simulink model "Modelo9"  (R2020b)
settings: Solver=FixedStepAuto  StartTime=0.0  StopTime=inf  FixedStep=1e-2  MaxStep=1e-4  RelTol=1e-3
model workspace (MAT data in the model file):
  sensor_carga = Simulink.Parameter
  sensor_carga.DataType = 'auto'
  sensor_carga.Dimensions = [0 0]
values from neighbouring files (symbols this model uses):
  bcx = 1000e3    (= 1000000)    [Datos_simulacion.m]
  bcy = 500e3    (= 500000)    [Datos_simulacion.m]
  beq_tc = (bv_c+beq_cel)/Rw^2    (= 27000)    [Datos_simulacion.m]
  beq_ti = (b_h+beq_iel)/Rd^2    (= 28800)    [Datos_simulacion.m]
  bw = 30e3    (= 30000)    [Datos_simulacion.m]
  g = 9.80665    [Datos_simulacion.m]
  i_c = 15    [Datos_simulacion.m]
  i_i = 30    [Datos_simulacion.m]
  Kcd = Meq_c*polo_c*n    (= 472500)    [Datos_simulacion.m]
  Kci = Kcp*polo_c/n    (= 1938936.66179)    [Datos_simulacion.m]
  Kcp = Kcd*polo_c    (= 1513396.48861)    [Datos_simulacion.m]
  Kcy = 1.3e9    (= 1300000000)    [Datos_simulacion.m]
  Kid = Kcp*polo_i/n    (= 1815537.84919)    [Datos_simulacion.m]
  Kii = Meq_i*polo_i*n    (= 360000)    [Datos_simulacion.m]
  Kip = Kcd*polo_i    (= 1417080.12441)    [Datos_simulacion.m]
  Kw = 1800e3    (= 1800000)    [Datos_simulacion.m]
  Meq_c = m_c+Jeq_c/Rw^2    (= 59008)    [Datos_simulacion.m]
  Meq_i = m_h+Jeq_i/Rd^2    (= 48014.2222222)    [Datos_simulacion.m]
  Rd = 0.75    [Datos_simulacion.m]
  Rw = 0.5    [Datos_simulacion.m]
  Tau = 1e-3    (= 0.001)    [Datos_simulacion.m]
libraries: simulink x2, pid_lib x1, fuzblock x1, dspswit3 x1
(part 1 of 2)
settings Model: PauseTimes=6  Creator=GoniR  LastModifiedBy=GoniR
settings SolverCC: ConcurrentTasks=on  ZeroCrossAlgorithm=Adaptive  AutoInsertRateTranBlk=on
settings DebuggingCC: MaskedZcDiagnostic=none  IgnoredZcDiagnostic=none
settings HardwareCC: ProdHWDeviceType=AMD->x86-64 (Windows64)
settings SFSimCC: SimTargetLang=C++
settings ConfigComp: PLC_TargetIDE=codesys23

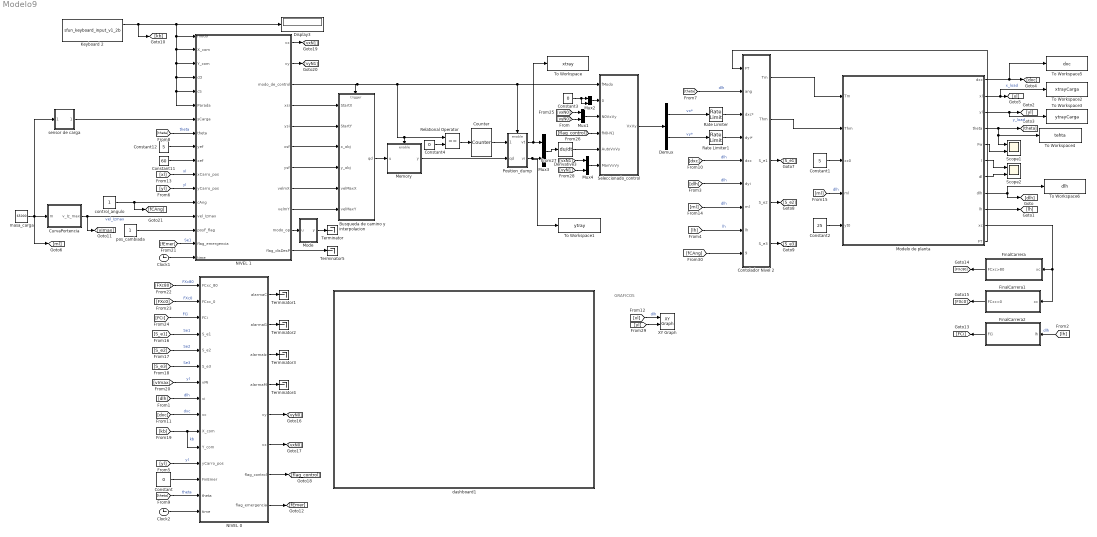
== system Modelo9 ==
  note: GRAFICOS
  Busqueda de camino y interpolacion : Subsystem
  Clock1 : Clock
  Clock2 : Clock
  Constant : Constant  Value=0
  Constant1 : Constant  Value=5
  Constant11 : Constant  Value=60
  Constant12 : Constant  Value=5
  Constant2 : Constant  Value=25
  Constant3 : Constant  Value=0
  Constant4 : Constant  Value=0
  Contolador Nivel 2 : Subsystem
  Counter : dspswit3/Counter  Direction=Up  CountEvent=Free running  CounterSize=User defined  MaxCount=100000  InitialCount=0  Output=Count  HitValue=32  ResetInput=on  SamplesPerFrame=1  Ts=-1  CntDtype=double  HitDtype=Logical
  CurvaPortencia : MATLAB Function  TreatAsAtomicUnit=on
  Demux : Demux  Outputs=2
  Derivative3 : Derivative
  Display3 : Display
  FinalCarrera : Subsystem
  FinalCarrera1 : Subsystem
  FinalCarrera2 : Subsystem
  Keyboard 2 : M-S-Function  FunctionName=sfun_keyboard_input_v1_2b  mask(Keyboard Input){}
      mask help: Keyboard Input
      mask Display: fprintf('Keyboard');
  Memory : Subsystem
  Mode : MATLAB Function  TreatAsAtomicUnit=on
  Modelo de planta : Subsystem
  Mux{1..4} (4 alike) : Mux  Inputs=2
  NIVEL 0 : Stateflow chart  TreatAsAtomicUnit=on
      settings: PortSchema="{\"entries\":[{\"content\":{\"sides\":[{\"content\":{\"connectorIds\":[\"In1\",\"In2\",\"In3\",\"In4\",\"In5\",\"In6\",\"In7\",\"In8\",\"In9\",\"In11\",\"In12\",\"In13\",\"In14\",\"In15\",\"In10\"]},\"type\":\"ConnectorPlacement.EquallySpacedRectSide\",\"uuid\":\"257bd8b2-e50d-4f94-a780-554a728b2489\"},{\"content\":{\"connectorIds\":[\"Out1\",\"Out2\",\"Out3\",\"Out4\",\"Out5\",\"Out6\",\"Out7\",\"Out8\"],\"side\":\"RIGHT\"},\"type\":\"ConnectorPlacement.EquallySpacedRectSide\",\"uuid\":\"e3415bb4-ca91-4503-b89e-6184bd1dfb63\"},{\"content\":{\"connectorIds\":[],\"side\":\"TOP\"},\"type\":\"ConnectorPlacement.EquallySpacedRectSide\",\"uuid\":\"9a32744b-d02f-467d-83f2-39baa82bdd9b\"},{\"content\":{\"connectorIds\":[],\"side\":\"HIDDEN\"},\"type\":\"ConnectorPlacement.EquallySpacedRectSide\",\"uuid\":\"21a6614f-2711-4cba-b5d3-48b2ed3c7fdc\"}]},\"type\":\"ConnectorPlacement.EquallySpacedConnector\",\"uuid\":\"64bd3217-fe30-40b0-9b87-0656394712b6\"}],\"packageUris\":[\"http://schema.mathworks.com/mf0/Connector/R2020b\"],\"version\":\"1.0\"}"
  NIVEL 1 : Stateflow chart  TreatAsAtomicUnit=on
      settings: PortSchema="{\"entries\":[{\"content\":{\"sides\":[{\"content\":{\"connectorIds\":[\"In13\",\"In1\",\"In2\",\"In5\",\"In6\",\"In10\",\"In7\",\"In14\",\"In3\",\"In4\",\"In9\",\"In12\",\"In8\",\"In15\",\"In17\",\"In16\",\"In11\"]},\"type\":\"ConnectorPlacement.EquallySpacedRectSide\",\"uuid\":\"1e4dd542-1771-4859-b91f-fc1cb250280a\"},{\"content\":{\"connectorIds\":[\"Out1\",\"Out2\",\"Out9\",\"Out7\",\"Out6\",\"Out8\",\"Out5\",\"Out4\",\"Out3\",\"Out10\",\"Out11\"],\"side\":\"RIGHT\"},\"type\":\"ConnectorPlacement.EquallySpacedRectSide\",\"uuid\":\"bb5e6521-c449-4a1c-9147-094c14f63665\"},{\"content\":{\"connectorIds\":[],\"side\":\"TOP\"},\"type\":\"ConnectorPlacement.EquallySpacedRectSide\",\"uuid\":\"54352a45-add1-4eb7-bb1e-2f57d731739f\"},{\"content\":{\"connectorIds\":[],\"side\":\"HIDDEN\"},\"type\":\"ConnectorPlacement.EquallySpacedRectSide\",\"uuid\":\"3e291a91-093a-4ab5-80ab-be4d5a353953\"}]},\"type\":\"ConnectorPlacement.EquallySpacedConnector\",\"uuid\":\"db8c49e8-a9b8-459f-b7fa-0d865c8e3061\"}],\"packageUris\":[\"http://schema.mathworks.com/mf0/Connector/R2020b\"],\"version\":\"1.0\"}"
  Position_dump : Subsystem
  Rate Limiter : RateLimiter  RisingSlewLimit=2  FallingSlewLimit=-2  SampleTimeMode=inherited
  Rate Limiter1 : RateLimiter  RisingSlewLimit=2  FallingSlewLimit=-2  SampleTimeMode=inherited
  Relational Operator : RelationalOperator  Operator===  OutDataTypeStr=boolean  RndMeth=Simplest
  Scope1 : Scope  NumInputPorts=2
  Scope2 : Scope  NumInputPorts=2
  Seleccionado_control : Subsystem
  Terminator{,1..5} (6 alike) : Terminator
  To Workspace : ToWorkspace  VariableName=xtray  SampleTime=-1
  To Workspace1 : ToWorkspace  VariableName=ytray  SampleTime=-1
  To Workspace2 : ToWorkspace  VariableName=xtrayCarga  SampleTime=-1
  To Workspace3 : ToWorkspace  VariableName=ytrayCarga  SampleTime=-1
  To Workspace4 : ToWorkspace  VariableName=tehta  SaveFormat=Timeseries  SampleTime=-1
  To Workspace5 : ToWorkspace  VariableName=dxc  SaveFormat=Timeseries  SampleTime=-1
  To Workspace6 : ToWorkspace  VariableName=dlh  SaveFormat=Timeseries  SampleTime=-1
  XY Graph : simulink/Sinks/XY Graph  xmin=0  xmax=80  ymin=0  ymax=60  st=-1
  control_angulo : Constant
  dashboard1 : Subsystem
  masa_carga : Constant  Value=65000
  pos_cambiada : Constant
  sensor de carga : Subsystem
  wires:
  Modelo de planta/2(xl) -> To Workspace2/1, [xl]  "x_load"
  Modelo de planta/3(yl) -> To Workspace3/1, [yl]  "y_load"
  Modelo de planta/7(dl) -> Scope2/2
  Modelo de planta/6(l) -> Scope2/1
  Modelo de planta/5(Fw) -> Scope1/2
  masa_carga/1 -> CurvaPortencia/1(m), [ml], sensor de carga/1(In1)
  Constant1/1 -> Modelo de planta/3(xc0)
  Constant2/1 -> Modelo de planta/5(yt0)
  Modelo de planta/4(theta) -> Scope1/1, To Workspace4/1, [theta]
  Memory/1(y) -> Position_dump/2(qd)
  Busqueda de camino y interpolacion/1(qd) -> Memory/1(u)
  Keyboard 2/1 -> NIVEL 1/2(Y_com), NIVEL 1/10(Parada), NIVEL 1/6(cS), NIVEL 1/5(cD), NIVEL 1/1(X_com), NIVEL 1/13(modo), Display3/1, [kb]
  Clock1/1 -> NIVEL 1/11(time)
  Constant11/1 -> NIVEL 1/4(xef)
  Constant12/1 -> NIVEL 1/3(yef)
  NIVEL 1/4(velmX) -> Busqueda de camino y interpolacion/5(velMaxX)
  NIVEL 1/3(velmY) -> Busqueda de camino y interpolacion/6(velMaxY)
  NIVEL 1/7(xsi) -> Busqueda de camino y interpolacion/1(StartX)
  NIVEL 1/6(ysi) -> Busqueda de camino y interpolacion/2(StartY)
  NIVEL 1/8(xsf) -> Busqueda de camino y interpolacion/3(x_obj)
  Position_dump/2(vi) -> To Workspace1/1, Mux3/2
  Demux/2 -> Rate Limiter1/1  "vy*"
  Demux/1 -> Rate Limiter/1  "vx*"
  control_angulo/1 -> NIVEL 1/8(cAng), [fCAng]
  NIVEL 1/10(modo_op) -> Mode/1(u)
  CurvaPortencia/1(v_Iz_max) -> NIVEL 1/15(vel_Izmax), [vImax]  "vel_Izmax"
  sensor de carga/1(Out1) -> NIVEL 1/7(sCarga)
  pos_cambiada/1 -> NIVEL 1/17(posF_flag)
  Mode/1(y) -> Terminator/1
  NIVEL 1/9(modo_de_control) -> Relational Operator/1, Memory/Enable, Seleccionado_control/1(fModo), Position_dump/Enable, Busqueda de camino y interpolacion/Trigger
  NIVEL 1/5(ysf) -> Busqueda de camino y interpolacion/4(y_obj)
  Rate Limiter/1 -> Contolador Nivel 2/3(dxc*)
  Modelo de planta/1(dxc) -> To Workspace5/1, [dxc]
  Modelo de planta/8(dlh) -> [dlh], To Workspace6/1
  Modelo de planta/9(lh) -> [lh]
  Contolador Nivel 2/1(Tm) -> Modelo de planta/1(Tm)
  Contolador Nivel 2/2(Thm) -> Modelo de planta/2(Thm)
  Rate Limiter1/1 -> Contolador Nivel 2/4(dyi*)
  Modelo de planta/10(xc) -> FinalCarrera1/1(xc), FinalCarrera/1(xc)
  Clock2/1 -> NIVEL 0/10(time)
  NIVEL 0/1(alarmaC) -> Terminator1/1
  NIVEL 0/2(alarmaG) -> Terminator2/1
  NIVEL 0/3(alarmaIz) -> Terminator3/1
  NIVEL 0/4(alarmaM) -> Terminator4/1
  Mux3/1 -> Derivative3/1
  Constant/1 -> NIVEL 0/14(FinEmer)
  NIVEL 0/8(flag_emergencia) -> [fEmer]
  Constant3/1 -> Mux2/1, Mux2/2
  Position_dump/1(vt) -> To Workspace/1, Mux3/1
  Constant4/1 -> Relational Operator/2
  Relational Operator/1 -> Counter/1
  Counter/1 -> Position_dump/1(counter)
  [dlh] -> Contolador Nivel 2/6(dyi)  "dlh"
  [dlh] -> NIVEL 0/8(vi)  "dlh"
  [lh] -> FinalCarrera2/1(lh)  "dlh"
  [lh] -> Contolador Nivel 2/8(lh)  "lh"
  [yl] -> NIVEL 0/13(yCarro_pos)  "yl"
  [yl] -> NIVEL 1/12(yCarro_pos)  "yl"
  [theta] -> Contolador Nivel 2/2(ang)  "dlh"
  [theta] -> NIVEL 0/15(theta)  "theta"
  [dxc] -> Contolador Nivel 2/5(dxc)  "dlh"
  [dxc] -> NIVEL 0/9(vc)  "dxc"
  [xl] -> XY Graph/1  "dlh"
  [xl] -> NIVEL 1/9(xCarro_pos)  "xl"
  [ml] -> Contolador Nivel 2/7(ml)  "dlh"
  [ml] -> Modelo de planta/4(ml)  "dlh"
  Contolador Nivel 2/3(S_e1) -> [S_e1]
  Contolador Nivel 2/4(S_e2) -> [S_e2]
  Contolador Nivel 2/5(S_e3) -> [S_e3]
  [S_e1] -> NIVEL 0/4(S_e1)  "Se1"
  [S_e2] -> NIVEL 0/5(S_e2)  "Se2"
  [S_e3] -> NIVEL 0/6(S_e3)  "Se3"
  [theta] -> NIVEL 1/14(theta)  "theta"
  [kb] -> NIVEL 0/12(Y_com), NIVEL 0/11(X_com)  "kb"
  [vImax] -> NIVEL 0/7(vMi)  "yl"
  [fEmer] -> NIVEL 1/16(flag_emergencia)  "Se1"
  FinalCarrera2/1(FCi) -> [FCi]
  FinalCarrera1/1(FCxc<0) -> [FXc0]
  FinalCarrera/1(FCxc>80) -> [FXc80]
  [FCi] -> NIVEL 0/3(FCi)  "FCi"
  [FXc0] -> NIVEL 0/2(FCxc_0)  "FXc0"
  [FXc80] -> NIVEL 0/1(FCxc_80)  "FXc80"
  NIVEL 0/5(vy) -> [vyN0]
  NIVEL 0/6(vx) -> [vxN0]
  [vyN0] -> Mux1/2
  [vxN0] -> Mux1/1
  NIVEL 0/7(flag_control) -> [flag_control]
  NIVEL 1/1(vx) -> [vxN1]
  NIVEL 1/2(vy) -> [vyN1]
  [vxN1] -> Mux4/1
  [vyN1] -> Mux4/2
  Mux2/1 -> Seleccionado_control/2(0)
  Mux1/1 -> Seleccionado_control/3(N0VxVy)
  [flag_control] -> Seleccionado_control/4(fN0-N1)
  Derivative3/1 -> Seleccionado_control/5(AutoVxVy)
  Mux4/1 -> Seleccionado_control/6(ManVxVy)
  Seleccionado_control/1(VxVy) -> Demux/1
  [yl] -> XY Graph/2
  NIVEL 1/11(flag_disDesP) -> Terminator5/1
  [fCAng] -> Contolador Nivel 2/9(fCAng)
  Modelo de planta/11(FT) -> Contolador Nivel 2/1(FT)

== system Modelo9/Busqueda de camino y interpolacion ==
  StartX : Inport
  StartY : Inport  Port=2
  x_obj : Inport  Port=3
  y_obj : Inport  Port=4
  velMaxX : Inport  Port=5
  velMaxY : Inport  Port=6
  Trigger : TriggerPort  VariantControl=Variant  PortDimensions=1
  Astart : MATLAB Function  TreatAsAtomicUnit=on
  Interpolador : MATLAB Function  TreatAsAtomicUnit=on
  qd : Outport
  wires:
  StartX/1 -> Astart/1(StartX)
  y_obj/1 -> Astart/4(y_obj)
  x_obj/1 -> Astart/3(x_obj)
  StartY/1 -> Astart/2(StartY)
  Astart/1(OptimalPath2) -> Interpolador/1(wayPoints)
  velMaxX/1 -> Interpolador/2(velMaxX)
  velMaxY/1 -> Interpolador/3(velMaxY)
  Interpolador/1(q) -> qd/1

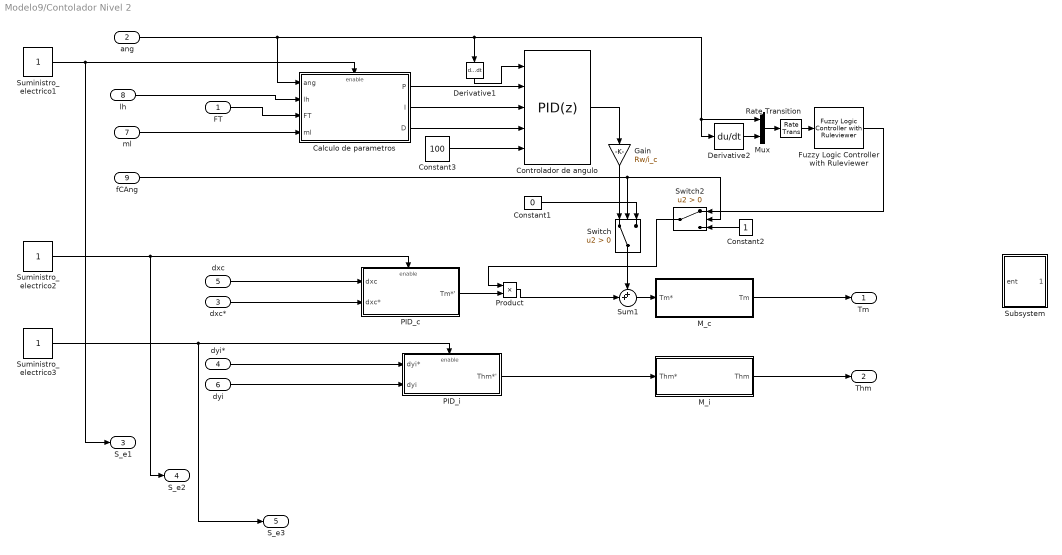
== system Modelo9/Contolador Nivel 2 ==
  FT : Inport
  ang : Inport  Port=2
  dxc* : Inport  Port=3
  dyi* : Inport  Port=4
  dxc : Inport  Port=5
  dyi : Inport  Port=6
  ml : Inport  Port=7
  lh : Inport  Port=8
  fCAng : Inport  Port=9
  Calculo de parametros : Subsystem
  Constant1 : Constant  Value=0
  Constant2 : Constant
  Constant3 : Constant  Value=100
  Controlador de angulo : pid_lib/PID Controller  Controller=PID  Form=Parallel  TimeDomain=Discrete-time  UseExternalTs=off  SampleTime=0.01  IntegratorMethod=Forward Euler  FilterMethod=Forward Euler  ControllerParametersSource=external  P=1  I=1  D=0  UseFilter=on  N=100  TunerSelectOption=Transfer Function Based (PID Tuner App)  InitialConditionSource=internal  InitialConditionForIntegrator=0  InitialConditionForFilter=0  DifferentiatorICPrevScaledInput=0  ExternalReset=none  TrackingMode=off  Kt=1  LimitOutput=off  SatLimitsSource=internal  UpperSaturationLimit=inf  LowerSaturationLimit=-inf  LinearizeAsGain=on  AntiWindupMode=none  Kb=1  POutMin=[]  POutMax=[]  IOutMin=[]  IOutMax=[]  DOutMin=[]  DOutMax=[]  NOutMin=[]  NOutMax=[]  SumOutMin=[]  SumOutMax=[]  SaturationOutMin=[]  SaturationOutMax=[]  PParamMin=[]  PParamMax=[]  IParamMin=[]  IParamMax=[]  DParamMin=[]  DParamMax=[]  NParamMin=[]  NParamMax=[]  KbParamMin=[]  KbParamMax=[]  KtParamMin=[]  KtParamMax=[]  KbOutMin=[]  KbOutMax=[]  KtOutMin=[]  KtOutMax=[]  IntegratorOutMin=[]  IntegratorOutMax=[]  FilterOutMin=[]  FilterOutMax=[]  SumI1OutMin=[]  SumI1OutMax=[]  SumI2OutMin=[]  SumI2OutMax=[]  SumI3OutMin=[]  SumI3OutMax=[]  SumI4OutMin=[]  SumI4OutMax=[]  SumDOutMin=[]  SumDOutMax=[]  DifferentiatorOutMin=[]  DifferentiatorOutMax=[]  FilterDiffOutCoefMin=[]  FilterDiffOutCoefMax=[]  ReciprocalOutMin=[]  ReciprocalOutMax=[]  SumDenOutMin=[]  SumDenOutMax=[]  SumNumOutMin=[]  SumNumOutMax=[]  DivideOutMin=[]  DivideOutMax=[]  UdiffTsProdOutMin=[]  UdiffTsProdOutMax=[]  NTsProdOutMin=[]  NTsProdOutMax=[]  UintegralTsProdOutMin=[]  UintegralTsProdOutMax=[]  UngainTsProdOutMin=[]  UngainTsProdOutMax=[]  IntegratorContinuousStateAttributes=''  IntegratorStateMustResolveToSignalObject=off  IntegratorRTWStateStorageClass=Auto  FilterContinuousStateAttributes=''  FilterStateMustResolveToSignalObject=off  FilterRTWStateStorageClass=Auto  ParallelPVariant=ExternalParameters  IdealPVariant=Disabled  IVariant=ExternalParameters  DVariant=ExternalParameters  IntegratorVariant=Discrete  SatVariant=Disabled  AWVariant=Passthrough  PCopyVariant=Disabled  TRVariant=Disabled  FdbkBlocksVariant=Forward  IdealPFdbkVariant=Disabled  SatFdbkVariant=Disabled  DerivativeFilterVariant=ForwardEulerFilter  NVariant=ExternalParameters  NCopyVariant=Disabled  FilterICVariant=InternalICsFilter  IntegratorICVariant=InternalICs  ExternalResetVariant=Disabled  TRSumVariant=Passthrough  SumFdbkVariant=Disabled  SumVariant=Sum_PID  TsampFilterVariant=InternalTs  TsampNgainVariant=Passthrough  TsampIntegralVariant=Passthrough  ExternalSaturationOutDataTypeStr=Inherit: Same as second input
  Derivative1 : Derivative
  Derivative2 : Derivative
  Fuzzy Logic Controller with Ruleviewer : fuzblock/Fuzzy Logic  Controller  with Ruleviewer  fismatrix=Control2  Ts=0.5
  Gain : Gain  Gain=Rw/i_c
  M_c : Subsystem
  M_i : Subsystem
  Mux : Mux  Inputs=2
  PID_c : Subsystem
  PID_i : Subsystem
  Product : Product
  Rate Transition : RateTransition  OutPortSampleTime=0.01
  Subsystem : Subsystem
  Sum1 : Sum  Inputs=++|
  Suministro_electrico1 : Constant
  Suministro_electrico2 : Constant
  Suministro_electrico3 : Constant
  Switch : Switch  Criteria=u2 > Threshold
  Switch2 : Switch  Criteria=u2 > Threshold
  Tm : Outport
  Thm : Outport  Port=2
  S_e1 : Outport  Port=3
  S_e2 : Outport  Port=4
  S_e3 : Outport  Port=5
  wires:
  Constant3/1 -> Controlador de angulo/5
  Fuzzy Logic Controller with Ruleviewer/1 -> Switch2/1
  Rate Transition/1 -> Fuzzy Logic Controller with Ruleviewer/1
  M_i/1(Thm) -> Thm/1
  Calculo de parametros/1(P) -> Controlador de angulo/2
  PID_i/1(Thm*') -> M_i/1(Thm*)
  Calculo de parametros/3(D) -> Controlador de angulo/4
  Calculo de parametros/2(I) -> Controlador de angulo/3
  ml/1 -> Calculo de parametros/4(ml)
  Mux/1 -> Rate Transition/1
  PID_c/1(Tm*') -> Product/2
  Sum1/1 -> M_c/1(Tm*)
  M_c/1(Tm) -> Tm/1
  dxc*/1 -> PID_c/2(dxc*)
  lh/1 -> Calculo de parametros/2(lh)
  dyi*/1 -> PID_i/1(dyi*)
  dxc/1 -> PID_c/1(dxc)
  dyi/1 -> PID_i/2(dyi)
  Derivative2/1 -> Mux/2
  Suministro_electrico1/1 -> S_e1/1, Calculo de parametros/Enable
  Suministro_electrico3/1 -> PID_i/Enable, S_e3/1
  Suministro_electrico2/1 -> S_e2/1, PID_c/Enable
  Switch/1 -> Sum1/1
  fCAng/1 -> Switch2/2, Switch/2
  Constant1/1 -> Switch/3
  Controlador de angulo/1 -> Gain/1
  Constant2/1 -> Switch2/3
  Switch2/1 -> Product/1
  Product/1 -> Sum1/2
  FT/1 -> Calculo de parametros/3(FT)
  Gain/1 -> Switch/1
  ang/1 -> Derivative2/1, Mux/1, Derivative1/1, Calculo de parametros/1(ang)
  Derivative1/1 -> Controlador de angulo/1

== system Modelo9/FinalCarrera ==
  xc : Inport
  Constant : Constant
  Constant1 : Constant  Value=0
  Switch : Switch  Criteria=u2 > Threshold  Threshold=80
  FCxc>80 : Outport
  wires:
  Constant/1 -> Switch/1
  Constant1/1 -> Switch/3
  Switch/1 -> FCxc>80/1
  xc/1 -> Switch/2

== system Modelo9/FinalCarrera1 ==
  xc : Inport
  Constant : Constant
  Constant1 : Constant  Value=0
  Gain : Gain  Gain=-1
  Switch : Switch  Criteria=u2 > Threshold
  FCxc<0 : Outport
  wires:
  Constant/1 -> Switch/1
  Constant1/1 -> Switch/3
  Switch/1 -> FCxc<0/1
  xc/1 -> Gain/1
  Gain/1 -> Switch/2

== system Modelo9/FinalCarrera2 ==
  lh : Inport
  Constant : Constant
  Constant1 : Constant  Value=0
  Gain : Gain  Gain=-1
  Switch : Switch
  FCi : Outport
  wires:
  Constant/1 -> Switch/1
  Constant1/1 -> Switch/3
  Switch/1 -> FCi/1
  lh/1 -> Gain/1
  Gain/1 -> Switch/2

== system Modelo9/Memory ==
  u : Inport
  Enable : EnablePort
  y : Outport
  wires:
  u/1 -> y/1

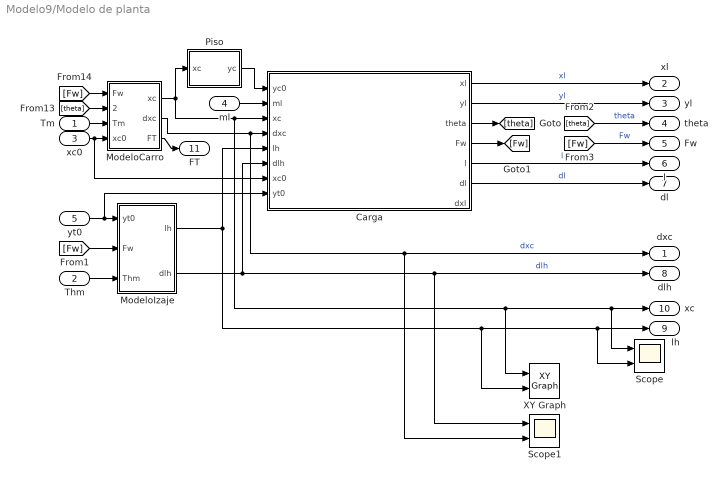
== system Modelo9/Modelo de planta ==
  Tm : Inport
  Thm : Inport  Port=2
  xc0 : Inport  Port=3
  ml : Inport  Port=4
  yt0 : Inport  Port=5
  Carga : Subsystem
  ModeloCarro : Subsystem
  ModeloIzaje : Subsystem
  Piso : Subsystem
  Scope : Scope  NumInputPorts=2
  Scope1 : Scope  NumInputPorts=2
  XY Graph : simulink/Sinks/XY Graph  xmin=0  xmax=80  ymin=0  ymax=60  st=-1
  dxc : Outport
  xl : Outport  Port=2
  yl : Outport  Port=3
  theta : Outport  Port=4
  Fw : Outport  Port=5
  l : Outport  Port=6
  dl : Outport  Port=7
  dlh : Outport  Port=8
  lh : Outport  Port=9
  xc : Outport  Port=10
  FT : Outport  Port=11
  wires:
  ModeloCarro/1(xc) -> XY Graph/1, Scope/1, xc/1, Carga/3(xc), Piso/1(xc)
  ModeloCarro/2(dxc) -> Scope1/2, dxc/1, Carga/4(dxc)  "dxc"
  ModeloIzaje/1(lh) -> XY Graph/2, Scope/2, lh/1, Carga/5(lh)
  ModeloIzaje/2(dlh) -> Carga/6(dlh), Scope1/1, dlh/1  "dlh"
  Carga/4(Fw) -> [Fw]
  [Fw] -> ModeloCarro/1(Fw)
  [Fw] -> ModeloIzaje/2(Fw)
  Carga/3(theta) -> [theta]
  [theta] -> ModeloCarro/2(theta)
  Carga/1(xl) -> xl/1  "xl"
  Carga/2(yl) -> yl/1  "yl"
  Carga/5(l) -> l/1  "l"
  Carga/6(dl) -> dl/1  "dl"
  [theta] -> theta/1  "theta"
  [Fw] -> Fw/1  "Fw"
  ml/1 -> Carga/2(ml)
  Thm/1 -> ModeloIzaje/3(Thm)
  Tm/1 -> ModeloCarro/3(Tm)
  Piso/1(yc) -> Carga/1(yc0)
  yt0/1 -> Carga/8(yt0), ModeloIzaje/1(yt0)
  xc0/1 -> Carga/7(xc0), ModeloCarro/4(xc0)
  ModeloCarro/3(FT) -> FT/1

== system Modelo9/Position_dump ==
  counter : Inport
  qd : Inport  Port=2
  Enable : EnablePort  PropagateVarSize=During execution
  MATLAB Function : MATLAB Function  TreatAsAtomicUnit=on
  Rate Transition : RateTransition
  Scope1 : Scope
  vt : Outport
  vi : Outport  Port=2
  wires:
  MATLAB Function/1(vt) -> vt/1
  MATLAB Function/2(vi) -> vi/1
  qd/1 -> MATLAB Function/1(qd)
  Rate Transition/1 -> Scope1/1, MATLAB Function/2(cont_i)
  counter/1 -> Rate Transition/1

== system Modelo9/Seleccionado_control ==
  fModo : Inport
  0 : Inport  Port=2
  N0VxVy : Inport  Port=3
  fN0-N1 : Inport  Port=4
  AutoVxVy : Inport  Port=5
  ManVxVy : Inport  Port=6
  AutoOn/Off : Switch  Criteria=u2 > Threshold
  M_o_A : Switch  Criteria=u2 > Threshold
  N0_o_N1 : Switch  Criteria=u2 > Threshold
  VxVy : Outport
  wires:
  AutoOn/Off/1 -> M_o_A/1
  N0_o_N1/1 -> VxVy/1
  M_o_A/1 -> N0_o_N1/3
  ManVxVy/1 -> M_o_A/3
  AutoVxVy/1 -> AutoOn/Off/1
  fModo/1 -> AutoOn/Off/2, M_o_A/2
  0/1 -> AutoOn/Off/3
  fN0-N1/1 -> N0_o_N1/2
  N0VxVy/1 -> N0_o_N1/1

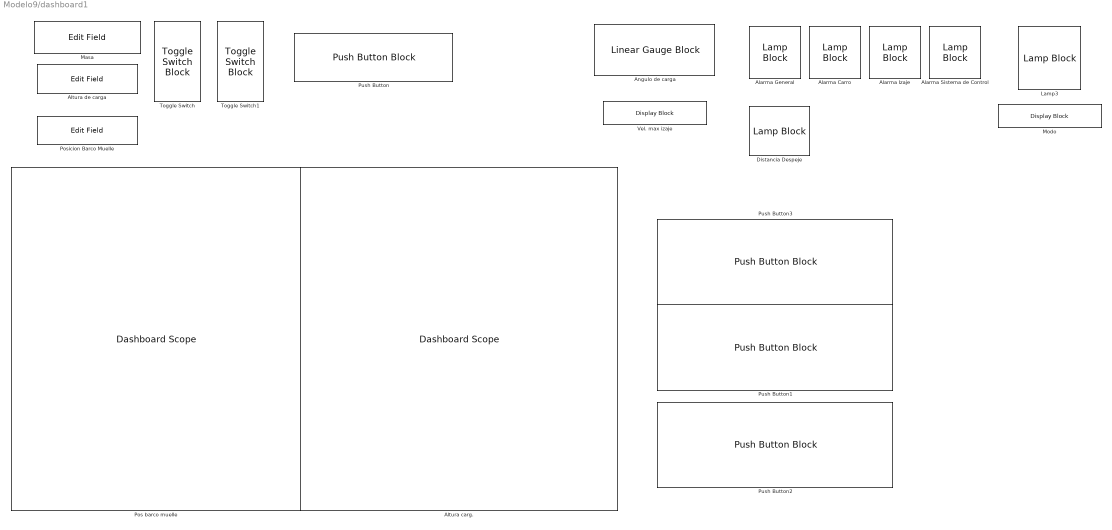
== system Modelo9/dashboard1 ==
  Alarma Carro : LampBlock
  Alarma General : LampBlock
  Alarma Izaje : LampBlock
  Alarma Sistema de Control : LampBlock
  Altura carg. : DashboardScope
  Altura de carga : EditField  LabelPosition=Hide  ShowInitialText=on  Alignment=Center
  Angulo de carga : LinearGaugeBlock  LabelPosition=Hide  ScaleMin=-0.15  ScaleMax=0.15
  Distancia Despeje : LampBlock
  Lamp3 : LampBlock  LabelPosition=Bottom
  Masa : EditField  LabelPosition=Hide  ShowInitialText=on  Alignment=Center
  Modo : DisplayBlock  LabelPosition=Hide  Format=short  Transparency=1
  Pos barco muelle : DashboardScope
  Posicion Barco Muelle : EditField  LabelPosition=Hide  ShowInitialText=on  Alignment=Center
  Push Button : PushButtonBlock  ButtonText=Fin Emergencia
  Push Button1 : PushButtonBlock  ButtonText=Falla Microcontrolador1  OnValue=0
  Push Button2 : PushButtonBlock  ButtonText=Falla Microcontrolador3  OnValue=0
  Push Button3 : PushButtonBlock  ButtonText=Falla Microcontrolador2  OnValue=0
  Toggle Switch : ToggleSwitchBlock
      settings: Values={{'Off', 'On'}, [0 1]}
  Toggle Switch1 : ToggleSwitchBlock
      settings: Values={{'Sin Cambiar', 'Cambiada'}, [0 1]}
  Vel. max izaje : DisplayBlock  LabelPosition=Hide  Format=short  Transparency=1

== system Modelo9/sensor de carga ==
  In1 : Inport
  Constant5 : Constant
  Constant6 : Constant  Value=0
  Switch1 : Switch  Criteria=u2 > Threshold  Threshold=15000
  Out1 : Outport
  wires:
  Constant5/1 -> Switch1/1
  Constant6/1 -> Switch1/3
  Switch1/1 -> Out1/1
  In1/1 -> Switch1/2

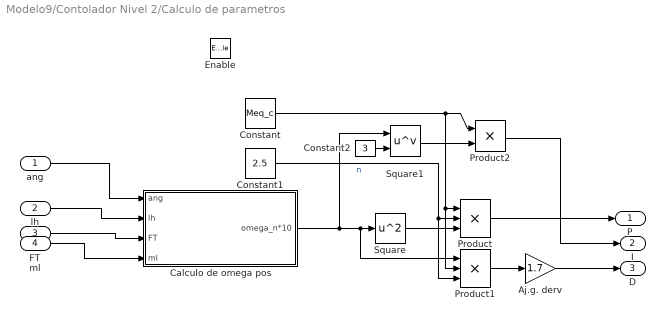
== system Modelo9/Contolador Nivel 2/Calculo de parametros ==
  ang : Inport
  lh : Inport  Port=2
  FT : Inport  Port=3
  ml : Inport  Port=4
  Enable : EnablePort
  Aj.g. derv : Gain  Gain=1.7
  Calculo de omega pos : Subsystem
  Constant : Constant  Value=Meq_c
  Constant1 : Constant  Value=2.5
  Constant2 : Constant  Value=3
  Product : Product  Inputs=3
  Product1 : Product  Inputs=3
  Product2 : Product
  Square : Math  Operator=square  SaturateOnIntegerOverflow=on
  Square1 : Math  Operator=pow  SaturateOnIntegerOverflow=on
  P : Outport
  I : Outport  Port=2
  D : Outport  Port=3
  wires:
  lh/1 -> Calculo de omega pos/2(lh)
  Constant1/1 -> Product/2, Product1/3  "n"
  Calculo de omega pos/1(omega_n*10) -> Square1/1, Product1/1, Square/1
  Constant/1 -> Product1/2, Product/1, Product2/1
  Product/1 -> P/1
  Product1/1 -> Aj.g. derv/1
  Square/1 -> Product/3
  ml/1 -> Calculo de omega pos/4(ml)
  Product2/1 -> I/1
  Aj.g. derv/1 -> D/1
  Square1/1 -> Product2/2
  Constant2/1 -> Square1/2
  FT/1 -> Calculo de omega pos/3(FT)
  ang/1 -> Calculo de omega pos/1(ang)

== system Modelo9/Contolador Nivel 2/M_c ==
  Tm* : Inport
  Transfer Fcn : TransferFcn  Denominator=[0.05 1]
  Tm : Outport
  wires:
  Tm*/1 -> Transfer Fcn/1
  Transfer Fcn/1 -> Tm/1

== system Modelo9/Contolador Nivel 2/M_i ==
  Thm* : Inport
  Transfer Fcn : TransferFcn  Denominator=[Tau 1]
  Thm : Outport
  wires:
  Thm*/1 -> Transfer Fcn/1
  Transfer Fcn/1 -> Thm/1

== system Modelo9/Contolador Nivel 2/PID_c ==
  dxc : Inport
  dxc* : Inport  Port=2
  Enable : EnablePort
  Gain : Gain  Gain=Kcp
  Gain1 : Gain  Gain=Kci
  Gain2 : Gain  Gain=Kcd
  Integrator : Integrator
  Integrator1 : Integrator
  Sum : Sum  Inputs=|+-
  Sum1 : Sum  Inputs=+++
  Tm*' : Outport
  wires:
  dxc*/1 -> Sum/1
  dxc/1 -> Sum/2
  Sum1/1 -> Tm*'/1
  Gain2/1 -> Sum1/3
  Gain/1 -> Sum1/2
  Gain1/1 -> Sum1/1
  Sum/1 -> Integrator1/1, Gain2/1
  Integrator1/1 -> Integrator/1, Gain/1
  Integrator/1 -> Gain1/1

== system Modelo9/Contolador Nivel 2/PID_i ==
  dyi* : Inport
  dyi : Inport  Port=2
  Enable : EnablePort
  Gain : Gain  Gain=Kip
  Gain1 : Gain  Gain=Kii
  Gain2 : Gain  Gain=Kid
  Integrator : Integrator
  Integrator1 : Integrator
  Sum : Sum  Inputs=|+-
  Sum1 : Sum  Inputs=+++
  Thm*' : Outport
  wires:
  dyi*/1 -> Sum/1
  dyi/1 -> Sum/2
  Sum1/1 -> Thm*'/1
  Gain2/1 -> Sum1/3
  Gain/1 -> Sum1/2
  Gain1/1 -> Sum1/1
  Sum/1 -> Integrator/1, Gain2/1
  Integrator/1 -> Integrator1/1, Gain/1
  Integrator1/1 -> Gain1/1

== system Modelo9/Contolador Nivel 2/Subsystem ==
  ent : Inport
  5secTimer : Subsystem
  Delay : Delay
  inv : Subsystem
  timer : Outport
  wires:
  ent/1 -> inv/1(ent)
  inv/1(inv) -> Delay/1, 5secTimer/Enable
  5secTimer/1(Out1) -> timer/1
  Delay/1 -> 5secTimer/1(In1)

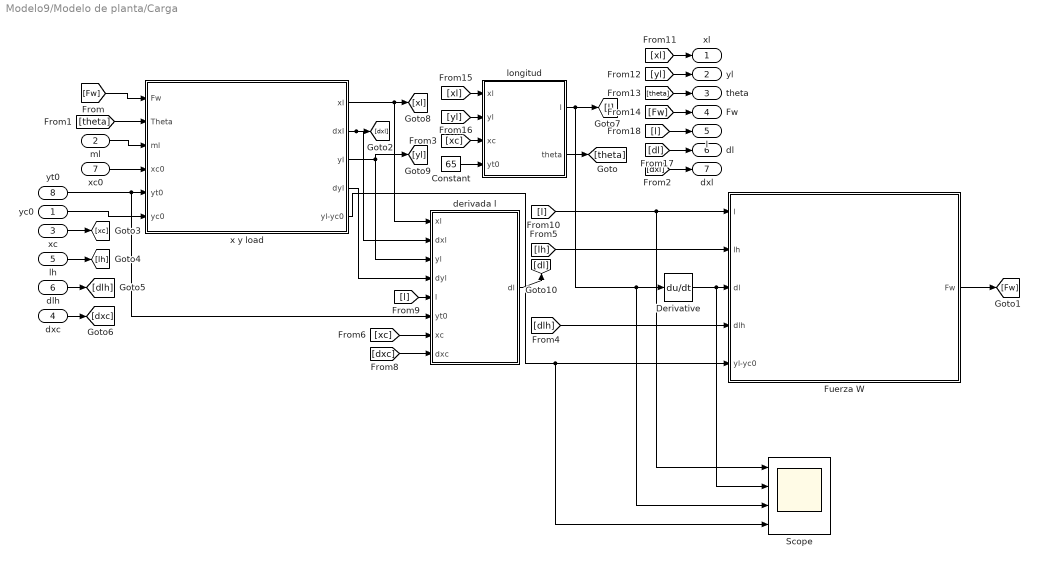
== system Modelo9/Modelo de planta/Carga ==
  yc0 : Inport
  ml : Inport  Port=2
  xc : Inport  Port=3
  dxc : Inport  Port=4
  lh : Inport  Port=5
  dlh : Inport  Port=6
  xc0 : Inport  Port=7
  yt0 : Inport  Port=8
  Constant : Constant  Value=65
  Derivative : Derivative
  Fuerza W : Subsystem
  Scope : Scope  NumInputPorts=4
  derivada l : Subsystem
  longitud : Subsystem
  x y load : Subsystem
  xl : Outport
  yl : Outport  Port=2
  theta : Outport  Port=3
  Fw : Outport  Port=4
  l : Outport  Port=5
  dl : Outport  Port=6
  dxl : Outport  Port=7
  wires:
  x y load/3(yl) -> [yl], derivada l/3(yl)
  derivada l/1(dl) -> [dl]
  longitud/2(theta) -> [theta]
  Fuerza W/1(Fw) -> [Fw]
  [theta] -> x y load/2(Theta)
  [Fw] -> x y load/1(Fw)
  ml/1 -> x y load/3(ml)
  yc0/1 -> x y load/6(yc0)
  xc/1 -> [xc]
  [xc] -> longitud/3(xc)
  lh/1 -> [lh]
  dlh/1 -> [dlh]
  [lh] -> Fuerza W/2(lh)
  [dlh] -> Fuerza W/4(dlh)
  x y load/1(xl) -> [xl], derivada l/1(xl)
  x y load/2(dxl) -> derivada l/2(dxl), [dxl]
  x y load/4(dyl) -> derivada l/4(dyl)
  dxc/1 -> [dxc]
  longitud/1(l) -> Scope/3, Derivative/1, [l]
  [l] -> Fuerza W/1(l), Scope/1
  [xl] -> xl/1
  [yl] -> yl/1
  [theta] -> theta/1
  [Fw] -> Fw/1
  [xl] -> longitud/1(xl)
  [yl] -> longitud/2(yl)
  [dl] -> dl/1
  [l] -> l/1
  [l] -> derivada l/5(l)
  [xc] -> derivada l/7(xc)
  [dxc] -> derivada l/8(dxc)
  x y load/5(yl-yc0) -> Scope/4, Fuerza W/5(yl-yc0)
  xc0/1 -> x y load/4(xc0)
  [dxl] -> dxl/1
  Constant/1 -> longitud/4(yt0)
  yt0/1 -> derivada l/6(yt0), x y load/5(yt0)
  Derivative/1 -> Scope/2, Fuerza W/3(dl)

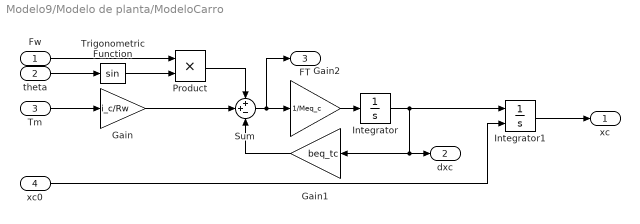
== system Modelo9/Modelo de planta/ModeloCarro ==
  Fw : Inport
  theta : Inport  Port=2
  Tm : Inport  Port=3
  xc0 : Inport  Port=4
  Gain : Gain  Gain=i_c/Rw
  Gain1 : Gain  Gain=beq_tc
  Gain2 : Gain  Gain=1/Meq_c
  Integrator : Integrator
  Integrator1 : Integrator  InitialConditionSource=external  InitialCondition=0.01
  Product : Product
  Sum : Sum  Inputs=++-
  Trigonometric Function : Trigonometry
  xc : Outport
  dxc : Outport  Port=2
  FT : Outport  Port=3
  wires:
  Product/1 -> Sum/1
  Integrator1/1 -> xc/1
  Gain2/1 -> Integrator/1
  Fw/1 -> Product/1
  Gain1/1 -> Sum/3
  Integrator/1 -> Integrator1/1, dxc/1, Gain1/1
  Tm/1 -> Gain/1
  Trigonometric Function/1 -> Product/2
  Sum/1 -> FT/1, Gain2/1
  theta/1 -> Trigonometric Function/1
  Gain/1 -> Sum/2
  xc0/1 -> Integrator1/2

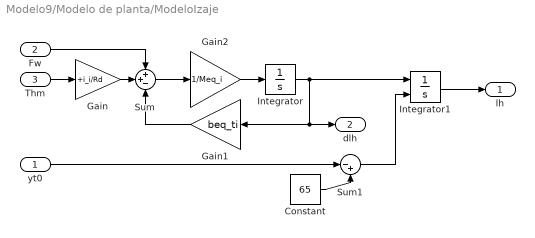
== system Modelo9/Modelo de planta/ModeloIzaje ==
  yt0 : Inport
  Fw : Inport  Port=2
  Thm : Inport  Port=3
  Constant : Constant  Value=65
  Gain : Gain  Gain=+i_i/Rd
  Gain1 : Gain  Gain=beq_ti
  Gain2 : Gain  Gain=1/Meq_i
  Integrator : Integrator
  Integrator1 : Integrator  InitialConditionSource=external  InitialCondition=0.5
  Sum : Sum  Inputs=++-
  Sum1 : Sum  Inputs=|-+
  lh : Outport
  dlh : Outport  Port=2
  wires:
  Fw/1 -> Sum/1
  Integrator1/1 -> lh/1
  Gain2/1 -> Integrator/1
  Gain1/1 -> Sum/3
  Integrator/1 -> Integrator1/1, Gain1/1, dlh/1
  Thm/1 -> Gain/1
  Sum/1 -> Gain2/1
  Gain/1 -> Sum/2
  Sum1/1 -> Integrator1/2
  yt0/1 -> Sum1/1
  Constant/1 -> Sum1/2

== system Modelo9/Modelo de planta/Piso ==
  xc : Inport
  Constant : Constant  Value=0
  yc : Outport
  wires:
  Constant/1 -> yc/1

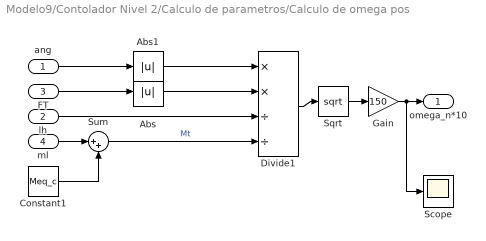
== system Modelo9/Contolador Nivel 2/Calculo de parametros/Calculo de omega pos ==
  ang : Inport
  lh : Inport  Port=2
  FT : Inport  Port=3
  ml : Inport  Port=4
  Abs : Abs
  Abs1 : Abs
  Constant1 : Constant  Value=Meq_c
  Divide1 : Product  Inputs=**//
  Gain : Gain  Gain=150
  Scope : Scope
  Sqrt : Sqrt  SaturateOnIntegerOverflow=on
  Sum : Sum  Inputs=|++
  omega_n*10 : Outport
  wires:
  Sqrt/1 -> Gain/1
  Divide1/1 -> Sqrt/1
  ml/1 -> Sum/1
  Constant1/1 -> Sum/2
  Gain/1 -> omega_n*10/1, Scope/1
  lh/1 -> Divide1/3
  FT/1 -> Abs/1
  ang/1 -> Abs1/1
  Sum/1 -> Divide1/4  "Mt"
  Abs1/1 -> Divide1/1
  Abs/1 -> Divide1/2

== system Modelo9/Contolador Nivel 2/Subsystem/5secTimer ==
  In1 : Inport
  Enable : EnablePort
  Constant : Constant  Value=0
  Constant1 : Constant
  Constant4 : Constant  Value=0
  Integrator : Integrator  ExternalReset=falling  InitialConditionSource=external
  Step : Step  Time=0  SampleTime=0
  Switch1 : Switch  Criteria=u2 > Threshold  Threshold=10
  Out1 : Outport
  wires:
  Constant4/1 -> Integrator/3
  Step/1 -> Integrator/1
  In1/1 -> Integrator/2
  Switch1/1 -> Out1/1
  Integrator/1 -> Switch1/2
  Constant1/1 -> Switch1/1
  Constant/1 -> Switch1/3

== system Modelo9/Contolador Nivel 2/Subsystem/inv ==
  ent : Inport
  Constant5 : Constant
  Constant6 : Constant  Value=0
  Switch1 : Switch  Criteria=u2 > Threshold
  inv : Outport
  wires:
  Constant6/1 -> Switch1/1
  Constant5/1 -> Switch1/3
  Switch1/1 -> inv/1
  ent/1 -> Switch1/2

== system Modelo9/Modelo de planta/Carga/Fuerza W ==
  l : Inport
  lh : Inport  Port=2
  dl : Inport  Port=3
  dlh : Inport  Port=4
  yl-yc0 : Inport  Port=5
  Gain : Gain  Gain=Kw
  Gain1 : Gain  Gain=0
  Gain2 : Gain  Gain=bw
  Sum : Sum  Inputs=|+-
  Sum1 : Sum  Inputs=|+-
  Sum2 : Sum  Inputs=|++
  Switch : Switch  Criteria=u2 > Threshold
  Fw : Outport
  wires:
  yl-yc0/1 -> Switch/2
  l/1 -> Sum/1
  lh/1 -> Sum/2
  Sum/1 -> Gain1/1, Gain/1
  Gain/1 -> Switch/1
  Gain1/1 -> Switch/3
  dl/1 -> Sum1/1
  dlh/1 -> Sum1/2
  Sum1/1 -> Gain2/1
  Switch/1 -> Sum2/1
  Gain2/1 -> Sum2/2
  Sum2/1 -> Fw/1

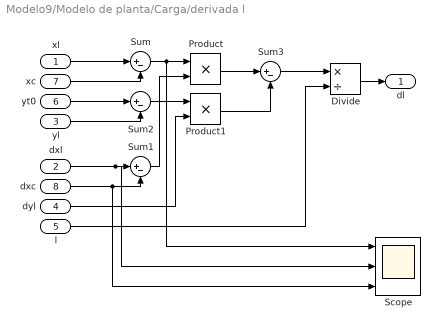
== system Modelo9/Modelo de planta/Carga/derivada l ==
  xl : Inport
  dxl : Inport  Port=2
  yl : Inport  Port=3
  dyl : Inport  Port=4
  l : Inport  Port=5
  yt0 : Inport  Port=6
  xc : Inport  Port=7
  dxc : Inport  Port=8
  Divide : Product  Inputs=*/
  Product : Product
  Product1 : Product
  Scope : Scope  NumInputPorts=3
  Sum{,1..3} (4 alike) : Sum  Inputs=|+-
  dl : Outport
  wires:
  xl/1 -> Sum/1
  xc/1 -> Sum/2
  dxl/1 -> Scope/2, Sum1/1
  dxc/1 -> Scope/3, Sum1/2
  Sum/1 -> Scope/1, Product/1
  Sum1/1 -> Product/2
  yt0/1 -> Sum2/1
  yl/1 -> Sum2/2
  dyl/1 -> Product1/2
  Sum2/1 -> Product1/1
  Product/1 -> Sum3/1
  Product1/1 -> Sum3/2
  Sum3/1 -> Divide/1
  Divide/1 -> dl/1
  l/1 -> Divide/2

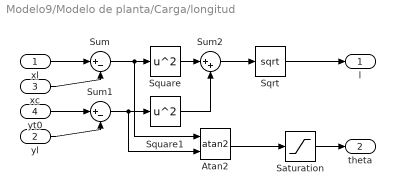
== system Modelo9/Modelo de planta/Carga/longitud ==
  xl : Inport
  yl : Inport  Port=2
  xc : Inport  Port=3
  yt0 : Inport  Port=4
  Atan2 : Trigonometry  Operator=atan2
  Saturation : Saturate  UpperLimit=pi/2  LowerLimit=-pi/2
  Sqrt : Sqrt  OutputSignalType=real  SaturateOnIntegerOverflow=on
  Square : Math  Operator=square  OutputSignalType=real  SaturateOnIntegerOverflow=on
  Square1 : Math  Operator=square  OutputSignalType=real  SaturateOnIntegerOverflow=on
  Sum : Sum  Inputs=|+-
  Sum1 : Sum  Inputs=|+-
  Sum2 : Sum  Inputs=|++
  l : Outport
  theta : Outport  Port=2
  wires:
  xl/1 -> Sum/1
  xc/1 -> Sum/2
  Sum/1 -> Atan2/1, Square/1
  yt0/1 -> Sum1/1
  yl/1 -> Sum1/2
  Sum1/1 -> Atan2/2, Square1/1
  Square/1 -> Sum2/1
  Square1/1 -> Sum2/2
  Sum2/1 -> Sqrt/1
  Atan2/1 -> Saturation/1
  Saturation/1 -> theta/1
  Sqrt/1 -> l/1

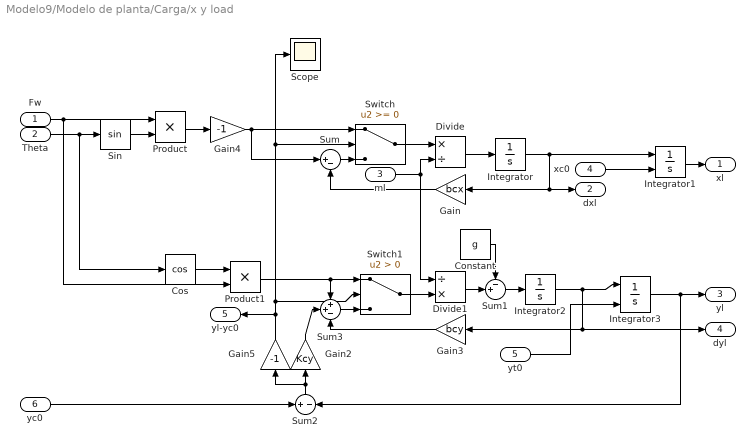
== system Modelo9/Modelo de planta/Carga/x y load ==
  Fw : Inport
  Theta : Inport  Port=2
  ml : Inport  Port=3
  xc0 : Inport  Port=4
  yt0 : Inport  Port=5
  yc0 : Inport  Port=6
  Constant : Constant  Value=g
  Cos : Trigonometry  Operator=cos
  Divide : Product  Inputs=*/
  Divide1 : Product  Inputs=/*
  Gain : Gain  Gain=bcx
  Gain2 : Gain  Gain=Kcy
  Gain3 : Gain  Gain=bcy
  Gain4 : Gain  Gain=-1
  Gain5 : Gain  Gain=-1
  Integrator : Integrator  ZeroCross=off
  Integrator1 : Integrator  InitialConditionSource=external  InitialCondition=0.01
  Integrator2 : Integrator
  Integrator3 : Integrator  InitialConditionSource=external  InitialCondition=1
  Product : Product
  Product1 : Product
  Scope : Scope
  Sin : Trigonometry
  Sum : Sum  Inputs=|+-
  Sum1 : Sum  Inputs=-+|
  Sum2 : Sum  Inputs=+-
  Sum3 : Sum  Inputs=++-
  Switch : Switch
  Switch1 : Switch  Criteria=u2 > Threshold
  xl : Outport
  dxl : Outport  Port=2
  yl : Outport  Port=3
  dyl : Outport  Port=4
  yl-yc0 : Outport  Port=5
  wires:
  Fw/1 -> Product/1, Product1/2
  Theta/1 -> Sin/1, Cos/1
  Sin/1 -> Product/2
  Product/1 -> Gain4/1
  Integrator/1 -> dxl/1, Gain/1, Integrator1/1
  Sum/1 -> Switch/3
  Gain/1 -> Sum/2
  Switch/1 -> Divide/1
  Divide/1 -> Integrator/1
  ml/1 -> Divide1/1, Divide/2
  Integrator1/1 -> xl/1
  Cos/1 -> Product1/1
  Product1/1 -> Sum3/1, Switch1/1
  Switch1/1 -> Divide1/2
  Integrator2/1 -> Gain3/1, dyl/1, Integrator3/1
  Integrator3/1 -> yl/1, Sum2/2
  Sum2/1 -> Gain5/1, Gain2/1
  yc0/1 -> Sum2/1
  Sum3/1 -> Switch1/3
  Gain2/1 -> Sum3/2
  Gain3/1 -> Sum3/3
  Gain4/1 -> Sum/1, Switch/1
  Gain5/1 -> yl-yc0/1, Scope/1, Switch/2, Switch1/2
  xc0/1 -> Integrator1/2
  yt0/1 -> Integrator3/2
  ? -> ?
  Constant/1 -> Sum1/1
  Divide1/1 -> Sum1/2
  Sum1/1 -> Integrator2/1

== stateflow chart Modelo9/NIVEL 1 ==
  state Nivel1
    state Spreder [parallel]
      settings: executionOrder=1
      state Descargado
        en:
        Scargado=0
      state Cargado
        en:
        Scargado=1
      (default) -> Descargado
      Descargado -> Cargado : [sCarga==1]
      Cargado -> Descargado : [sCarga==0]
    state controlAngulo [parallel]
      settings: executionOrder=2
      state Desactivado
      state Activado
      (default) -> Activado
      Activado -> Desactivado : [cAng==0]
      Desactivado -> Activado : [cAng==1]
    state modoOperacion [parallel]
      settings: executionOrder=3
      state Automatico
        state CicloSimple
          state descaragBarco
            en :
            xsi=xCarro_pos;
            ysi=yCarro_pos;
            xsf=xef;
            ysf=yef;
            velmX=4;
            velmY=vel_Izmax
            modo_de_control=1
            du:
            error=Calc_error(xsf,xCarro_pos,ysf,yCarro_pos);
          state cargaBarco
            en :
            xsi=xCarro_pos;
            ysi=yCarro_pos;
            xsf=xef;
            ysf=yef;
            velmX=4;
            velmY=vel_Izmax;
            modo_de_control=1;
            du:
            error=Calc_error(xsf,xCarro_pos,ysf,yCarro_pos);
          state standby
            en :
            modo_op = 2;
          state idaBarco
            en :
            xsi=xCarro_pos;
            ysi=yCarro_pos;
            xsf=xef;
            ysf=yef;
            velmX=4;
            velmY=vel_Izmax;
            modo_de_control=1;
            du:
            error=Calc_error(xsf,xCarro_pos,ysf,yCarro_pos);
          state vueltaMuelle
            en :
            xsi=xCarro_pos
            ysi=yCarro_pos
            xsf=xef
            ysf=yef
            velmX=4
            velmY=vel_Izmax
            modo_de_control=1
            du:
            error=Calc_error(xsf,xCarro_pos,ysf,yCarro_pos);
          Nivel1.modoOperacion.Automatico.CicloSimple.standby -> Nivel1.modoOperacion.Automatico.CicloSimple.cargaBarco [order 1] : [Scargado==1 && xCarro_pos<30 ]
          Nivel1.modoOperacion.Automatico.CicloSimple.standby -> Nivel1.modoOperacion.Automatico.CicloSimple.descaragBarco [order 2] : [Scargado==1 && xCarro_pos>30]
          (default) -> Nivel1.modoOperacion.Automatico.CicloSimple.standby
          Nivel1.modoOperacion.Automatico.CicloSimple.standby -> vueltaMuelle [order 3] : [Scargado==0 && xCarro_pos>30]
          Nivel1.modoOperacion.Automatico.CicloSimple.standby -> idaBarco [order 4] : [Scargado==0 && xCarro_pos<30]
        state standby
          en:
          error=inf;
          modo_op = 1;
        state CicloDoble
          state cargaBarco
            en :
            xsi=xCarro_pos;
            ysi=yCarro_pos;
            xsf=xef;
            ysf=yef;
            velmX=4;
            velmY=vel_Izmax;
            error=inf;
            modo_de_control=1;
            flagD_cB=1;
            du :
            error=Calc_error(xsf,xCarro_pos,ysf,yCarro_pos);
          state standby
            en:
            modo_op = 3;
            flagcD=1;
            cont=cont+1;
            if(cont==2)
            flagcD=0;
            cont=0;
            end
          state descaragBarco
            en :
            xsi=xCarro_pos;
            ysi=yCarro_pos;
            xsf=xef;
            ysf=yef;
            velmX=4;
            velmY=vel_Izmax;
            error=inf;
            modo_de_control=1;
            flagD_cB=0;
            du:
            error=Calc_error(xsf,xCarro_pos,ysf,yCarro_pos);
          Nivel1.modoOperacion.Automatico.CicloDoble.standby -> Nivel1.modoOperacion.Automatico.CicloDoble.cargaBarco [order 1] : [xCarro_pos<30]
          (default) -> Nivel1.modoOperacion.Automatico.CicloDoble.standby
          Nivel1.modoOperacion.Automatico.CicloDoble.standby -> Nivel1.modoOperacion.Automatico.CicloDoble.descaragBarco [order 2] : [xCarro_pos>30]
        Nivel1.modoOperacion.Automatico.standby -> CicloSimple [order 1] : [cS==115 && posF_flag]
        CicloSimple -> Nivel1.modoOperacion.Automatico.standby : [Parada==112 ]
        (default) -> Nivel1.modoOperacion.Automatico.standby
        Nivel1.modoOperacion.Automatico.standby -> CicloDoble [order 2] : [(cD==100 && posF_flag)|| flagcD]
        CicloDoble -> Nivel1.modoOperacion.Automatico.standby : [Parada==112 ]
      state modoManual
        en :
        modo_op = 0;
        xsi=xCarro_pos;
        ysi=yCarro_pos;
        vx=0;
        vy=0;
        time_a=time;
        vx_a=0;
        vy_a=0;
        error=0;
        delta_t=0;
        modo_de_control=0;
        dist_desp=yCarro_pos-20;
        if(dist_desp>2)
        flag_disDesP=1;
        else
        flag_disDesP=0;
        end
        du :
        delta_t=time-time_a;
        [vx,vy]=Calc_v(delta_t,vx_a,vy_a,X_com,Y_com);
        time_a=time;
        vx_a=vx;
        vy_a=vy;
      state transicion
        en:
        time_a=time;
        delta_t=0;
        du:
        delta_t=time-time_a;
        [vx,vy]=Calc_v1(delta_t,vx,vy);
        time_a=time;
        ex:
        vx = 0;
        vy = 0;
      state transicion1
        en:
        time_a=time
        delta_t=0
        du:
        delta_t=time-time_a;
        [vx,vy]=Calc_v1(delta_t,vx,vy);
        time_a=time;
        ex:
        vx = 0
        vy = 0
      (default) -> modoManual
      transicion -> Automatico : [abs(vx)<0.1 && abs(vy)<0.01]
      modoManual -> transicion : [modo==97 && (dist_desp>2 || xCarro_pos>30)   ]
      Automatico -> transicion1 [order 1] : [error<2 && theta <0.05 || modo==109]
      transicion1 -> modoManual : [abs(vx)<0.1 && abs(vy)<0.01]
      Automatico -> transicion1 [order 2] : [flag_emergencia]
  (default) -> Nivel1
  data: delta_t2 function_input double; vx_a2 function_input double; vy_a2 function_input double; vx2 function_output; vy2 function_output; er function_output; xf function_input; xpos function_input; yf function_input; ypos function_input; delta_t1 function_input double; vx_a1 function_input double; vy_a1 function_input double; vx1 function_output; vy1 function_output; X_com1 function_input; Y_com1 function_input; X_com input; Y_com input; vx output; opManual local; vy output; yef input; xef input; velmY output; velmX output; ysf output; ysi output; xsi output; xsf output; cD input; Scargado local; cS input; sCarga input; cAng input; xCarro_pos input; Parada input; time input; time_i local; vx_a local; time_a local; yCarro_pos input; error local; vy_a local; delta_t local; modo input; modo_de_control output; flagD_cB local; cont local =0; theta input; dist_desp local; modo_op output; vel_Izmax input; flag_emergencia input; posF_flag input; flag_disDesP output; flagcD local =0
  function [vx2,vy2]=Calc_v1(delta_t2,vx_a2,vy_a2):
    | function [vx2,vy2]=Calc_v1(delta_t2,vx_a2,vy_a2)
    | if (vx_a2 < 0 )
    |     vx2=0.2*(delta_t2)+vx_a2;
    | else
    |     vx2=-0.2*(delta_t2)+vx_a2;
    | end
    | if (vy_a2 < 0)
    |     vy2=0.2*(delta_t2)+vy_a2;
    | else
    |     vy2=-0.2*(delta_t2)+vy_a2;
    | end
    | end
  function er=Calc_error(xf,xpos,yf,ypos):
    | function er=Calc_error(xf,xpos,yf,ypos)
    |     er=((xf-xpos)^2+(yf-ypos)^2)^0.5;
  function [vx1,vy1]=Calc_v(delta_t1,vx_a1,vy_a1,X_com1,Y_com1):
    | function [vx1,vy1]=Calc_v(delta_t1,vx_a1,vy_a1,X_com1,Y_com1)
    | if (X_com1 == 29 && vx_a1<4)
    |     vx1=0.8*(delta_t1)+vx_a1;
    | elseif (X_com1 == 28 && vx_a1 > -4 )
    |     vx1=-0.8*(delta_t1)+vx_a1;
    | else
    |     vx1=vx_a1;
    | end
    | if (Y_com1 == 31 && vy_a1<1.5)
    |     vy1=0.8*(delta_t1)+vy_a1;
    | elseif (Y_com1==30 && vy_a1>-1.5)
    |     vy1=-0.8*(delta_t1)+vy_a1;
    | else
    |     vy1=vy_a1;
    | end
    | 
    | end

== matlab function Modelo9/CurvaPortencia ==
  data: m input; v_Iz_max output
function v_Iz_max  = calc_vmax(m)

p = 956150;

v_Iz_max = p/(m*9.8);

if v_Iz_max>3
    v_Iz_max=3;
    
end

== matlab function Modelo9/Busqueda de camino y interpolacion/Astart ==
  data: StartX input; StartY input; x_obj input; OptimalPath2 output size=2,100; y_obj input
function OptimalPath2=ASTARPATH(StartX,StartY,x_obj,y_obj)
%Version 1.0
% By Einar Ueland 2nd of May, 2016
%%%
StartX= round(StartX);
StartY= round(StartY);
dist_seg=2;
MAP=int8(zeros(60,80));
%%% Generating a MAP
%1 represent an object that the path cannot penetrate, zero is a free path
MAP(20,1:30)=1;
MAP(1:20,30)=1;
MAP(80:45,1)=1;
MAP(20:35+dist_seg,30-dist_seg:30+dist_seg)=1;
MAP(20:35+dist_seg,30-dist_seg:30+dist_seg)=1;
MAP(1:30,35)=1;
MAP(1:30,37)=1;
MAP(1:30,39)=1;
MAP(1:30,41)=1;
MAP(1:30,43)=1;
MAP(1:30,45)=1;
MAP(1:30,47)=1;
MAP(1:30,49)=1;
MAP(1:30,51)=1;
MAP(1:30,53)=1;
MAP(1:30,55)=1;

%Start Positions

plot(MAP);
%Generating goal nodes, which is represented by a matrix. Several goals can be speciefied, in which case the pathfinder will find the closest goal. 
%a cell with the value 1 represent a goal cell
GoalRegister=int8(zeros(60,80));
GoalRegister(y_obj,x_obj)=1;
%%%
Connecting_Distance=16;
%nNeighboor=3;
% Preallocation of Matrices
[Height,Width]=size(MAP); %Height and width of matrix
GScore=zeros(Height,Width);           %Matrix keeping track of G-scores 
FScore=single(inf(Height,Width));     %Matrix keeping track of F-scores (only open list) 
Hn=single(zeros(Height,Width));       %Heuristic matrix
OpenMAT=int8(zeros(Height,Width));    %Matrix keeping of open grid cells
ClosedMAT=int8(zeros(Height,Width));  %Matrix keeping track of closed grid cells
ClosedMAT(MAP==1)=1;                  %Adding object-cells to closed matrix
ParentX=zeros(Height,Width);   %Matrix keeping track of X position of parent
ParentY=zeros(Height,Width);   %Matrix keeping track of Y position of parent


%%% Setting up matrices representing neighboors to be investigated
NeighboorCheck=ones(2*Connecting_Distance+1);
Dummy=2*Connecting_Distance+2;
Mid=Connecting_Distance+1;
for i=1:Connecting_Distance-1
NeighboorCheck(i,i)=0;
NeighboorCheck(Dummy-i,i)=0;
NeighboorCheck(i,Dummy-i)=0;
NeighboorCheck(Dummy-i,Dummy-i)=0;
NeighboorCheck(Mid,i)=0;
NeighboorCheck(Mid,Dummy-i)=0;
NeighboorCheck(i,Mid)=0;
NeighboorCheck(Dummy-i,Mid)=0;
end
NeighboorCheck(Mid,Mid)=0;

[row, col]=find(NeighboorCheck==1);
Neighboors=[row col]-(Connecting_Distance+1);
N_Neighboors=size(col,1);
%%% End of setting up matrices representing neighboors to be investigated


%%%%%%%%% Creating Heuristic-matrix based on distance to nearest  goal node
[ row,col]=find(GoalRegister==1);
RegisteredGoals=[row col];
Nodesfound=size(RegisteredGoals,1);

for k=1:size(GoalRegister,1)
    for j=1:size(GoalRegister,2)
        if MAP(k,j)==0
            Mat=RegisteredGoals-(repmat([j k],(Nodesfound),1));
            Distance=(min(sqrt(sum(abs(Mat).^2,2))));
            Hn(k,j)=Distance;
        end
    end
end
%End of creating Heuristic-matrix. 

%Note: If Hn values is set to zero the method will reduce to the Dijkstras method.

%Initializign start node with FValue and opening first node.
FScore(StartY,StartX)=Hn(StartY,StartX);         
OpenMAT(StartY,StartX)=1;   
CurrentY=0;
CurrentX=0;


while 1==1 %Code will break when path found or when no path exist
    MINopenFSCORE=min(min(FScore));
    if MINopenFSCORE==inf;
    %Failuere!
    OptimalPath=[inf];
    RECONSTRUCTPATH=0;
     break
    end
    [CurrentY,CurrentX]=find(FScore==MINopenFSCORE);
    CurrentY=CurrentY(1);
    CurrentX=CurrentX(1);

    if GoalRegister(CurrentY,CurrentX)==1
    %GOAL!!
        RECONSTRUCTPATH=1;
        break
    end
    
  %Remobing node from OpenList to ClosedList  
    OpenMAT(CurrentY,CurrentX)=0;
    FScore(CurrentY,CurrentX)=inf;
    ClosedMAT(CurrentY,CurrentX)=1;
    for p=1:N_Neighboors
        i=Neighboors(p,1); %Y
        j=Neighboors(p,2); %X
        if CurrentY+i<1||CurrentY+i>Height||CurrentX+j<1||CurrentX+j>Width
            continue
        end
        Flag=1;
        if(ClosedMAT(CurrentY+i,CurrentX+j)==0) %Neiboor is open;
            if (abs(i)>1||abs(j)>1);   
                % Need to check that the path does not pass an object
                JumpCells=2*max(abs(i),abs(j))-1;
                for K=1:JumpCells;
                    YPOS=round(K*i/JumpCells);
                    XPOS=round(K*j/JumpCells);
            
                    if (MAP(CurrentY+YPOS,CurrentX+XPOS)==1)
                        Flag=0;
                    end
                end
            end
             %End of  checking that the path does not pass an object

            if Flag==1;           
                tentative_gScore = GScore(CurrentY,CurrentX) + sqrt(i^2+j^2);
                if OpenMAT(CurrentY+i,CurrentX+j)==0
                    OpenMAT(CurrentY+i,CurrentX+j)=1;                    
                elseif tentative_gScore >= GScore(CurrentY+i,CurrentX+j)
                    continue
                end
                ParentX(CurrentY+i,CurrentX+j)=CurrentX;
                ParentY(CurrentY+i,CurrentX+j)=CurrentY;
                GScore(CurrentY+i,CurrentX+j)=tentative_gScore;
                FScore(CurrentY+i,CurrentX+j)= tentative_gScore+Hn(CurrentY+i,CurrentX+j);
            end
        end
    end
end

k=2;
OptimalPath=zeros(100,2);
OptimalPath(:,:)=-1;
if RECONSTRUCTPATH
    OptimalPath(1,:)=[CurrentY CurrentX];
    while RECONSTRUCTPATH
        CurrentXDummy=ParentX(CurrentY,CurrentX);
        CurrentY=ParentY(CurrentY,CurrentX);
        CurrentX=CurrentXDummy;
        OptimalPath(k,:)=[CurrentY CurrentX];
        k=k+1;
        if (((CurrentX== StartX)) &&(CurrentY==StartY))
            break
        end
    end
end
contador=0;
for l=1:100
    if OptimalPath(l,1)~=-1
        contador=contador+1;
    end
end
OptimalPath=OptimalPath';
OptimalPath2=zeros(2,contador);
OptimalPath2=OptimalPath(:,1:contador);

end

== matlab function Modelo9/Mode ==
  data: u input; y output
function y = mode(u)
if u==0
y="manual";
elseif u==1
y="automatico";
elseif u==2
y="automatico_simple";
else  
y="automatico_doble";
end
